simulink model "simu"  (R2022b)
settings: Solver=VariableStepAuto  StartTime=0.0  StopTime=300  RelTol=1e-3
values from neighbouring files (symbols this model uses):
  den = [2153 1]    [controladorPID.m]
  Kcciclos = 1349.8    [controladorPID.m]
  Kph = 2.39 * 10^-4    (= 0.000239)    [controladorPID.m]
  Ksensor = 0.1    [controladorPID.m]
  num = 4899.2    [controladorPID.m]
  R = 16.129    [controladorPID.m]
undefined symbols (not defined in the file or in its folder): denC, numC
settings Model: Creator=cafes  LastModifiedBy=55499
settings DebuggingCC: UnconnectedInputMsg=warning  UnconnectedOutputMsg=warning  UnconnectedLineMsg=warning
settings ModelReferenceCC: EnableRefExpFcnMdlSchedulingChecks=on
settings RTWCC: DLArmComputeVersion=19.05

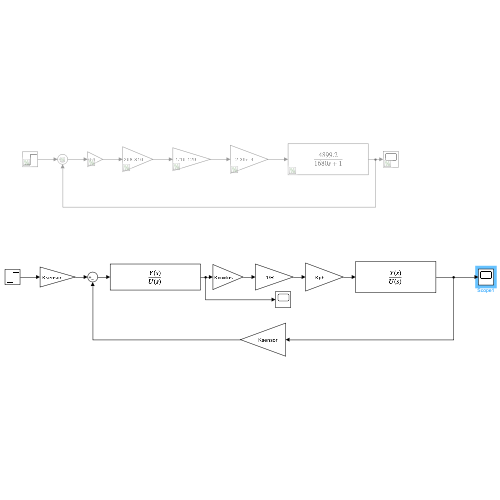
[thumbnail: Simulink's stored preview of the top-level diagram]
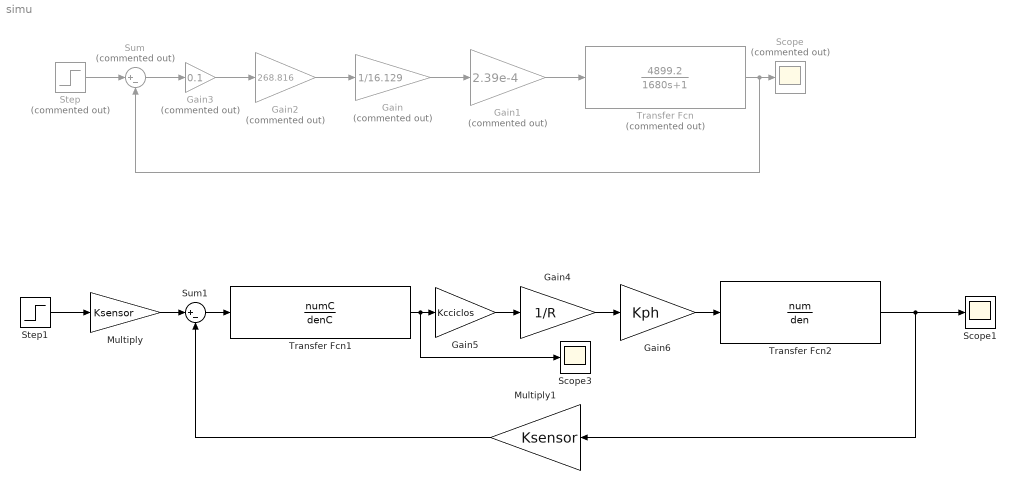
== system simu ==
  Gain : Gain  Commented=on  Gain=1/16.129
  Gain1 : Gain  Commented=on  Gain=2.39e-4
  Gain2 : Gain  Commented=on  Gain=268.816
  Gain3 : Gain  Commented=on  Gain=0.1
  Gain4 : Gain  Gain=1/R
  Gain5 : Gain  Gain=Kcciclos
  Gain6 : Gain  Gain=Kph
  Multiply : Gain  Gain=Ksensor
  Multiply1 : Gain  Gain=Ksensor
  Scope : Scope  Commented=on
  Scope1 : Scope
  Scope3 : Scope
  Step : Step  Commented=on  After=80  SampleTime=0
  Step1 : Step  Time=0  After=80  SampleTime=0
  Sum : Sum  Commented=on  Inputs=|+-
  Sum1 : Sum  Inputs=|+-
  Transfer Fcn : TransferFcn  Commented=on  Numerator=[4899.2]  Denominator=[1680 1]
  Transfer Fcn1 : TransferFcn  Numerator=numC  Denominator=denC
  Transfer Fcn2 : TransferFcn  Numerator=num  Denominator=den
  wires:
  Gain3/1 -> Gain2/1
  Gain2/1 -> Gain/1
  Sum/1 -> Gain3/1
  Transfer Fcn/1 -> Sum/2, Scope/1
  Gain1/1 -> Transfer Fcn/1
  Step/1 -> Sum/1
  Gain/1 -> Gain1/1
  Sum1/1 -> Transfer Fcn1/1
  Multiply/1 -> Sum1/1
  Transfer Fcn1/1 -> Scope3/1, Gain5/1
  Gain5/1 -> Gain4/1
  Gain4/1 -> Gain6/1
  Gain6/1 -> Transfer Fcn2/1
  Transfer Fcn2/1 -> Scope1/1, Multiply1/1
  Multiply1/1 -> Sum1/2
  Step1/1 -> Multiply/1
